simulink model "gm_MATE_HDLsolver_myFirstCircuit"  (R2024b)
settings: Solver=FixedStepDiscrete  StartTime=0.0  StopTime=0.05  FixedStep=6.02409638554217e-09  MaxStep=100e-6  RelTol=1e-4
PostLoadFcn:
  | Ts=1e-6; nb_sw=3; nb_lc=2;nb_r=1;nb_src=1; nb_out=3; rL=1.2;rC=100;L=1e-3; C=1e-5; LpejoSw=1e-6;h=Ts; MAX_INPUTS=16;
  | MAX_OUTPUTS=16;
  | MAX_SWITCHES=8;
  | MAX_INPUTS=16;
InitFcn:
  | Ts=1e-6; nb_sw=3; nb_lc=2;nb_r=1;nb_src=1; nb_out=3; rL=1.2;rC=100;L=1e-3; C=1e-5; LpejoSw=1e-6;h=Ts; MAX_INPUTS=16;
  | MAX_OUTPUTS=16;
  | MAX_SWITCHES=8;
  | MAX_INPUTS=16;
undefined symbols (not defined in the file or in its folder): MATE_SOC
libraries: fl_lib x31, nesl_utility x13, hdlmdlgenlib x10, simetranss x5, simulink x4, hdlsllib x3, ee_lib x2, eeGeneralControl x1
(part 6 of 8)

== system gm_MATE_HDLsolver_myFirstCircuit/ForFPGA/mul_Dot Product13_dotp_7 ==
  In1 : Inport
  In2 : Inport  Port=2
  mul_Dot Product13_dotp_7 : Product  Inputs=**  OutDataTypeStr=single  SampleTime=6.02409638554217e-09
  mul_Dot Product13_dotp_7_pd1 : Delay  DelayLength=6
  Out1 : Outport
  wires:
  In1/1 -> mul_Dot Product13_dotp_7/1
  In2/1 -> mul_Dot Product13_dotp_7/2
  mul_Dot Product13_dotp_7/1 -> mul_Dot Product13_dotp_7_pd1/1
  mul_Dot Product13_dotp_7_pd1/1 -> Out1/1

== system gm_MATE_HDLsolver_myFirstCircuit/ForFPGA/mul_Dot Product13_dotp_8 ==
  In1 : Inport
  In2 : Inport  Port=2
  mul_Dot Product13_dotp_8 : Product  Inputs=**  OutDataTypeStr=single  SampleTime=6.02409638554217e-09
  mul_Dot Product13_dotp_8_pd1 : Delay  DelayLength=6
  Out1 : Outport
  wires:
  In1/1 -> mul_Dot Product13_dotp_8/1
  In2/1 -> mul_Dot Product13_dotp_8/2
  mul_Dot Product13_dotp_8/1 -> mul_Dot Product13_dotp_8_pd1/1
  mul_Dot Product13_dotp_8_pd1/1 -> Out1/1

== system gm_MATE_HDLsolver_myFirstCircuit/ForFPGA/mul_Dot Product13_dotp_9 ==
  In1 : Inport
  In2 : Inport  Port=2
  mul_Dot Product13_dotp_9 : Product  Inputs=**  OutDataTypeStr=single  SampleTime=6.02409638554217e-09
  mul_Dot Product13_dotp_9_pd1 : Delay  DelayLength=6
  Out1 : Outport
  wires:
  In1/1 -> mul_Dot Product13_dotp_9/1
  In2/1 -> mul_Dot Product13_dotp_9/2
  mul_Dot Product13_dotp_9/1 -> mul_Dot Product13_dotp_9_pd1/1
  mul_Dot Product13_dotp_9_pd1/1 -> Out1/1

== system gm_MATE_HDLsolver_myFirstCircuit/ForFPGA/mul_Dot Product14_dotp_0 ==
  In1 : Inport
  In2 : Inport  Port=2
  mul_Dot Product14_dotp_0 : Product  Inputs=**  OutDataTypeStr=single  SampleTime=6.02409638554217e-09
  mul_Dot Product14_dotp_0_pd1 : Delay  DelayLength=6
  Out1 : Outport
  wires:
  In1/1 -> mul_Dot Product14_dotp_0/1
  In2/1 -> mul_Dot Product14_dotp_0/2
  mul_Dot Product14_dotp_0/1 -> mul_Dot Product14_dotp_0_pd1/1
  mul_Dot Product14_dotp_0_pd1/1 -> Out1/1

== system gm_MATE_HDLsolver_myFirstCircuit/ForFPGA/mul_Dot Product14_dotp_1 ==
  In1 : Inport
  In2 : Inport  Port=2
  mul_Dot Product14_dotp_1 : Product  Inputs=**  OutDataTypeStr=single  SampleTime=6.02409638554217e-09
  mul_Dot Product14_dotp_1_pd1 : Delay  DelayLength=6
  Out1 : Outport
  wires:
  In1/1 -> mul_Dot Product14_dotp_1/1
  In2/1 -> mul_Dot Product14_dotp_1/2
  mul_Dot Product14_dotp_1/1 -> mul_Dot Product14_dotp_1_pd1/1
  mul_Dot Product14_dotp_1_pd1/1 -> Out1/1

== system gm_MATE_HDLsolver_myFirstCircuit/ForFPGA/mul_Dot Product14_dotp_10 ==
  In1 : Inport
  In2 : Inport  Port=2
  mul_Dot Product14_dotp_10 : Product  Inputs=**  OutDataTypeStr=single  SampleTime=6.02409638554217e-09
  mul_Dot Product14_dotp_10_pd1 : Delay  DelayLength=6
  Out1 : Outport
  wires:
  In1/1 -> mul_Dot Product14_dotp_10/1
  In2/1 -> mul_Dot Product14_dotp_10/2
  mul_Dot Product14_dotp_10/1 -> mul_Dot Product14_dotp_10_pd1/1
  mul_Dot Product14_dotp_10_pd1/1 -> Out1/1

== system gm_MATE_HDLsolver_myFirstCircuit/ForFPGA/mul_Dot Product14_dotp_11 ==
  In1 : Inport
  In2 : Inport  Port=2
  mul_Dot Product14_dotp_11 : Product  Inputs=**  OutDataTypeStr=single  SampleTime=6.02409638554217e-09
  mul_Dot Product14_dotp_11_pd1 : Delay  DelayLength=6
  Out1 : Outport
  wires:
  In1/1 -> mul_Dot Product14_dotp_11/1
  In2/1 -> mul_Dot Product14_dotp_11/2
  mul_Dot Product14_dotp_11/1 -> mul_Dot Product14_dotp_11_pd1/1
  mul_Dot Product14_dotp_11_pd1/1 -> Out1/1

== system gm_MATE_HDLsolver_myFirstCircuit/ForFPGA/mul_Dot Product14_dotp_12 ==
  In1 : Inport
  In2 : Inport  Port=2
  mul_Dot Product14_dotp_12 : Product  Inputs=**  OutDataTypeStr=single  SampleTime=6.02409638554217e-09
  mul_Dot Product14_dotp_12_pd1 : Delay  DelayLength=6
  Out1 : Outport
  wires:
  In1/1 -> mul_Dot Product14_dotp_12/1
  In2/1 -> mul_Dot Product14_dotp_12/2
  mul_Dot Product14_dotp_12/1 -> mul_Dot Product14_dotp_12_pd1/1
  mul_Dot Product14_dotp_12_pd1/1 -> Out1/1

== system gm_MATE_HDLsolver_myFirstCircuit/ForFPGA/mul_Dot Product14_dotp_13 ==
  In1 : Inport
  In2 : Inport  Port=2
  mul_Dot Product14_dotp_13 : Product  Inputs=**  OutDataTypeStr=single  SampleTime=6.02409638554217e-09
  mul_Dot Product14_dotp_13_pd1 : Delay  DelayLength=6
  Out1 : Outport
  wires:
  In1/1 -> mul_Dot Product14_dotp_13/1
  In2/1 -> mul_Dot Product14_dotp_13/2
  mul_Dot Product14_dotp_13/1 -> mul_Dot Product14_dotp_13_pd1/1
  mul_Dot Product14_dotp_13_pd1/1 -> Out1/1

== system gm_MATE_HDLsolver_myFirstCircuit/ForFPGA/mul_Dot Product14_dotp_14 ==
  In1 : Inport
  In2 : Inport  Port=2
  mul_Dot Product14_dotp_14 : Product  Inputs=**  OutDataTypeStr=single  SampleTime=6.02409638554217e-09
  mul_Dot Product14_dotp_14_pd1 : Delay  DelayLength=6
  Out1 : Outport
  wires:
  In1/1 -> mul_Dot Product14_dotp_14/1
  In2/1 -> mul_Dot Product14_dotp_14/2
  mul_Dot Product14_dotp_14/1 -> mul_Dot Product14_dotp_14_pd1/1
  mul_Dot Product14_dotp_14_pd1/1 -> Out1/1

== system gm_MATE_HDLsolver_myFirstCircuit/ForFPGA/mul_Dot Product14_dotp_15 ==
  In1 : Inport
  In2 : Inport  Port=2
  mul_Dot Product14_dotp_15 : Product  Inputs=**  OutDataTypeStr=single  SampleTime=6.02409638554217e-09
  mul_Dot Product14_dotp_15_pd1 : Delay  DelayLength=6
  Out1 : Outport
  wires:
  In1/1 -> mul_Dot Product14_dotp_15/1
  In2/1 -> mul_Dot Product14_dotp_15/2
  mul_Dot Product14_dotp_15/1 -> mul_Dot Product14_dotp_15_pd1/1
  mul_Dot Product14_dotp_15_pd1/1 -> Out1/1

== system gm_MATE_HDLsolver_myFirstCircuit/ForFPGA/mul_Dot Product14_dotp_2 ==
  In1 : Inport
  In2 : Inport  Port=2
  mul_Dot Product14_dotp_2 : Product  Inputs=**  OutDataTypeStr=single  SampleTime=6.02409638554217e-09
  mul_Dot Product14_dotp_2_pd1 : Delay  DelayLength=6
  Out1 : Outport
  wires:
  In1/1 -> mul_Dot Product14_dotp_2/1
  In2/1 -> mul_Dot Product14_dotp_2/2
  mul_Dot Product14_dotp_2/1 -> mul_Dot Product14_dotp_2_pd1/1
  mul_Dot Product14_dotp_2_pd1/1 -> Out1/1

== system gm_MATE_HDLsolver_myFirstCircuit/ForFPGA/mul_Dot Product14_dotp_3 ==
  In1 : Inport
  In2 : Inport  Port=2
  mul_Dot Product14_dotp_3 : Product  Inputs=**  OutDataTypeStr=single  SampleTime=6.02409638554217e-09
  mul_Dot Product14_dotp_3_pd1 : Delay  DelayLength=6
  Out1 : Outport
  wires:
  In1/1 -> mul_Dot Product14_dotp_3/1
  In2/1 -> mul_Dot Product14_dotp_3/2
  mul_Dot Product14_dotp_3/1 -> mul_Dot Product14_dotp_3_pd1/1
  mul_Dot Product14_dotp_3_pd1/1 -> Out1/1

== system gm_MATE_HDLsolver_myFirstCircuit/ForFPGA/mul_Dot Product14_dotp_4 ==
  In1 : Inport
  In2 : Inport  Port=2
  mul_Dot Product14_dotp_4 : Product  Inputs=**  OutDataTypeStr=single  SampleTime=6.02409638554217e-09
  mul_Dot Product14_dotp_4_pd1 : Delay  DelayLength=6
  Out1 : Outport
  wires:
  In1/1 -> mul_Dot Product14_dotp_4/1
  In2/1 -> mul_Dot Product14_dotp_4/2
  mul_Dot Product14_dotp_4/1 -> mul_Dot Product14_dotp_4_pd1/1
  mul_Dot Product14_dotp_4_pd1/1 -> Out1/1

== system gm_MATE_HDLsolver_myFirstCircuit/ForFPGA/mul_Dot Product14_dotp_5 ==
  In1 : Inport
  In2 : Inport  Port=2
  mul_Dot Product14_dotp_5 : Product  Inputs=**  OutDataTypeStr=single  SampleTime=6.02409638554217e-09
  mul_Dot Product14_dotp_5_pd1 : Delay  DelayLength=6
  Out1 : Outport
  wires:
  In1/1 -> mul_Dot Product14_dotp_5/1
  In2/1 -> mul_Dot Product14_dotp_5/2
  mul_Dot Product14_dotp_5/1 -> mul_Dot Product14_dotp_5_pd1/1
  mul_Dot Product14_dotp_5_pd1/1 -> Out1/1

== system gm_MATE_HDLsolver_myFirstCircuit/ForFPGA/mul_Dot Product14_dotp_6 ==
  In1 : Inport
  In2 : Inport  Port=2
  mul_Dot Product14_dotp_6 : Product  Inputs=**  OutDataTypeStr=single  SampleTime=6.02409638554217e-09
  mul_Dot Product14_dotp_6_pd1 : Delay  DelayLength=6
  Out1 : Outport
  wires:
  In1/1 -> mul_Dot Product14_dotp_6/1
  In2/1 -> mul_Dot Product14_dotp_6/2
  mul_Dot Product14_dotp_6/1 -> mul_Dot Product14_dotp_6_pd1/1
  mul_Dot Product14_dotp_6_pd1/1 -> Out1/1

== system gm_MATE_HDLsolver_myFirstCircuit/ForFPGA/mul_Dot Product14_dotp_7 ==
  In1 : Inport
  In2 : Inport  Port=2
  mul_Dot Product14_dotp_7 : Product  Inputs=**  OutDataTypeStr=single  SampleTime=6.02409638554217e-09
  mul_Dot Product14_dotp_7_pd1 : Delay  DelayLength=6
  Out1 : Outport
  wires:
  In1/1 -> mul_Dot Product14_dotp_7/1
  In2/1 -> mul_Dot Product14_dotp_7/2
  mul_Dot Product14_dotp_7/1 -> mul_Dot Product14_dotp_7_pd1/1
  mul_Dot Product14_dotp_7_pd1/1 -> Out1/1

== system gm_MATE_HDLsolver_myFirstCircuit/ForFPGA/mul_Dot Product14_dotp_8 ==
  In1 : Inport
  In2 : Inport  Port=2
  mul_Dot Product14_dotp_8 : Product  Inputs=**  OutDataTypeStr=single  SampleTime=6.02409638554217e-09
  mul_Dot Product14_dotp_8_pd1 : Delay  DelayLength=6
  Out1 : Outport
  wires:
  In1/1 -> mul_Dot Product14_dotp_8/1
  In2/1 -> mul_Dot Product14_dotp_8/2
  mul_Dot Product14_dotp_8/1 -> mul_Dot Product14_dotp_8_pd1/1
  mul_Dot Product14_dotp_8_pd1/1 -> Out1/1

== system gm_MATE_HDLsolver_myFirstCircuit/ForFPGA/mul_Dot Product14_dotp_9 ==
  In1 : Inport
  In2 : Inport  Port=2
  mul_Dot Product14_dotp_9 : Product  Inputs=**  OutDataTypeStr=single  SampleTime=6.02409638554217e-09
  mul_Dot Product14_dotp_9_pd1 : Delay  DelayLength=6
  Out1 : Outport
  wires:
  In1/1 -> mul_Dot Product14_dotp_9/1
  In2/1 -> mul_Dot Product14_dotp_9/2
  mul_Dot Product14_dotp_9/1 -> mul_Dot Product14_dotp_9_pd1/1
  mul_Dot Product14_dotp_9_pd1/1 -> Out1/1

== system gm_MATE_HDLsolver_myFirstCircuit/ForFPGA/mul_Dot Product15_dotp_0 ==
  In1 : Inport
  In2 : Inport  Port=2
  mul_Dot Product15_dotp_0 : Product  Inputs=**  OutDataTypeStr=single  SampleTime=6.02409638554217e-09
  mul_Dot Product15_dotp_0_pd1 : Delay  DelayLength=6
  Out1 : Outport
  wires:
  In1/1 -> mul_Dot Product15_dotp_0/1
  In2/1 -> mul_Dot Product15_dotp_0/2
  mul_Dot Product15_dotp_0/1 -> mul_Dot Product15_dotp_0_pd1/1
  mul_Dot Product15_dotp_0_pd1/1 -> Out1/1

== system gm_MATE_HDLsolver_myFirstCircuit/ForFPGA/mul_Dot Product15_dotp_1 ==
  In1 : Inport
  In2 : Inport  Port=2
  mul_Dot Product15_dotp_1 : Product  Inputs=**  OutDataTypeStr=single  SampleTime=6.02409638554217e-09
  mul_Dot Product15_dotp_1_pd1 : Delay  DelayLength=6
  Out1 : Outport
  wires:
  In1/1 -> mul_Dot Product15_dotp_1/1
  In2/1 -> mul_Dot Product15_dotp_1/2
  mul_Dot Product15_dotp_1/1 -> mul_Dot Product15_dotp_1_pd1/1
  mul_Dot Product15_dotp_1_pd1/1 -> Out1/1

== system gm_MATE_HDLsolver_myFirstCircuit/ForFPGA/mul_Dot Product15_dotp_10 ==
  In1 : Inport
  In2 : Inport  Port=2
  mul_Dot Product15_dotp_10 : Product  Inputs=**  OutDataTypeStr=single  SampleTime=6.02409638554217e-09
  mul_Dot Product15_dotp_10_pd1 : Delay  DelayLength=6
  Out1 : Outport
  wires:
  In1/1 -> mul_Dot Product15_dotp_10/1
  In2/1 -> mul_Dot Product15_dotp_10/2
  mul_Dot Product15_dotp_10/1 -> mul_Dot Product15_dotp_10_pd1/1
  mul_Dot Product15_dotp_10_pd1/1 -> Out1/1

== system gm_MATE_HDLsolver_myFirstCircuit/ForFPGA/mul_Dot Product15_dotp_11 ==
  In1 : Inport
  In2 : Inport  Port=2
  mul_Dot Product15_dotp_11 : Product  Inputs=**  OutDataTypeStr=single  SampleTime=6.02409638554217e-09
  mul_Dot Product15_dotp_11_pd1 : Delay  DelayLength=6
  Out1 : Outport
  wires:
  In1/1 -> mul_Dot Product15_dotp_11/1
  In2/1 -> mul_Dot Product15_dotp_11/2
  mul_Dot Product15_dotp_11/1 -> mul_Dot Product15_dotp_11_pd1/1
  mul_Dot Product15_dotp_11_pd1/1 -> Out1/1

== system gm_MATE_HDLsolver_myFirstCircuit/ForFPGA/mul_Dot Product15_dotp_12 ==
  In1 : Inport
  In2 : Inport  Port=2
  mul_Dot Product15_dotp_12 : Product  Inputs=**  OutDataTypeStr=single  SampleTime=6.02409638554217e-09
  mul_Dot Product15_dotp_12_pd1 : Delay  DelayLength=6
  Out1 : Outport
  wires:
  In1/1 -> mul_Dot Product15_dotp_12/1
  In2/1 -> mul_Dot Product15_dotp_12/2
  mul_Dot Product15_dotp_12/1 -> mul_Dot Product15_dotp_12_pd1/1
  mul_Dot Product15_dotp_12_pd1/1 -> Out1/1

== system gm_MATE_HDLsolver_myFirstCircuit/ForFPGA/mul_Dot Product15_dotp_13 ==
  In1 : Inport
  In2 : Inport  Port=2
  mul_Dot Product15_dotp_13 : Product  Inputs=**  OutDataTypeStr=single  SampleTime=6.02409638554217e-09
  mul_Dot Product15_dotp_13_pd1 : Delay  DelayLength=6
  Out1 : Outport
  wires:
  In1/1 -> mul_Dot Product15_dotp_13/1
  In2/1 -> mul_Dot Product15_dotp_13/2
  mul_Dot Product15_dotp_13/1 -> mul_Dot Product15_dotp_13_pd1/1
  mul_Dot Product15_dotp_13_pd1/1 -> Out1/1

== system gm_MATE_HDLsolver_myFirstCircuit/ForFPGA/mul_Dot Product15_dotp_14 ==
  In1 : Inport
  In2 : Inport  Port=2
  mul_Dot Product15_dotp_14 : Product  Inputs=**  OutDataTypeStr=single  SampleTime=6.02409638554217e-09
  mul_Dot Product15_dotp_14_pd1 : Delay  DelayLength=6
  Out1 : Outport
  wires:
  In1/1 -> mul_Dot Product15_dotp_14/1
  In2/1 -> mul_Dot Product15_dotp_14/2
  mul_Dot Product15_dotp_14/1 -> mul_Dot Product15_dotp_14_pd1/1
  mul_Dot Product15_dotp_14_pd1/1 -> Out1/1

== system gm_MATE_HDLsolver_myFirstCircuit/ForFPGA/mul_Dot Product15_dotp_15 ==
  In1 : Inport
  In2 : Inport  Port=2
  mul_Dot Product15_dotp_15 : Product  Inputs=**  OutDataTypeStr=single  SampleTime=6.02409638554217e-09
  mul_Dot Product15_dotp_15_pd1 : Delay  DelayLength=6
  Out1 : Outport
  wires:
  In1/1 -> mul_Dot Product15_dotp_15/1
  In2/1 -> mul_Dot Product15_dotp_15/2
  mul_Dot Product15_dotp_15/1 -> mul_Dot Product15_dotp_15_pd1/1
  mul_Dot Product15_dotp_15_pd1/1 -> Out1/1

== system gm_MATE_HDLsolver_myFirstCircuit/ForFPGA/mul_Dot Product15_dotp_2 ==
  In1 : Inport
  In2 : Inport  Port=2
  mul_Dot Product15_dotp_2 : Product  Inputs=**  OutDataTypeStr=single  SampleTime=6.02409638554217e-09
  mul_Dot Product15_dotp_2_pd1 : Delay  DelayLength=6
  Out1 : Outport
  wires:
  In1/1 -> mul_Dot Product15_dotp_2/1
  In2/1 -> mul_Dot Product15_dotp_2/2
  mul_Dot Product15_dotp_2/1 -> mul_Dot Product15_dotp_2_pd1/1
  mul_Dot Product15_dotp_2_pd1/1 -> Out1/1

== system gm_MATE_HDLsolver_myFirstCircuit/ForFPGA/mul_Dot Product15_dotp_3 ==
  In1 : Inport
  In2 : Inport  Port=2
  mul_Dot Product15_dotp_3 : Product  Inputs=**  OutDataTypeStr=single  SampleTime=6.02409638554217e-09
  mul_Dot Product15_dotp_3_pd1 : Delay  DelayLength=6
  Out1 : Outport
  wires:
  In1/1 -> mul_Dot Product15_dotp_3/1
  In2/1 -> mul_Dot Product15_dotp_3/2
  mul_Dot Product15_dotp_3/1 -> mul_Dot Product15_dotp_3_pd1/1
  mul_Dot Product15_dotp_3_pd1/1 -> Out1/1

== system gm_MATE_HDLsolver_myFirstCircuit/ForFPGA/mul_Dot Product15_dotp_4 ==
  In1 : Inport
  In2 : Inport  Port=2
  mul_Dot Product15_dotp_4 : Product  Inputs=**  OutDataTypeStr=single  SampleTime=6.02409638554217e-09
  mul_Dot Product15_dotp_4_pd1 : Delay  DelayLength=6
  Out1 : Outport
  wires:
  In1/1 -> mul_Dot Product15_dotp_4/1
  In2/1 -> mul_Dot Product15_dotp_4/2
  mul_Dot Product15_dotp_4/1 -> mul_Dot Product15_dotp_4_pd1/1
  mul_Dot Product15_dotp_4_pd1/1 -> Out1/1

== system gm_MATE_HDLsolver_myFirstCircuit/ForFPGA/mul_Dot Product15_dotp_5 ==
  In1 : Inport
  In2 : Inport  Port=2
  mul_Dot Product15_dotp_5 : Product  Inputs=**  OutDataTypeStr=single  SampleTime=6.02409638554217e-09
  mul_Dot Product15_dotp_5_pd1 : Delay  DelayLength=6
  Out1 : Outport
  wires:
  In1/1 -> mul_Dot Product15_dotp_5/1
  In2/1 -> mul_Dot Product15_dotp_5/2
  mul_Dot Product15_dotp_5/1 -> mul_Dot Product15_dotp_5_pd1/1
  mul_Dot Product15_dotp_5_pd1/1 -> Out1/1

== system gm_MATE_HDLsolver_myFirstCircuit/ForFPGA/mul_Dot Product15_dotp_6 ==
  In1 : Inport
  In2 : Inport  Port=2
  mul_Dot Product15_dotp_6 : Product  Inputs=**  OutDataTypeStr=single  SampleTime=6.02409638554217e-09
  mul_Dot Product15_dotp_6_pd1 : Delay  DelayLength=6
  Out1 : Outport
  wires:
  In1/1 -> mul_Dot Product15_dotp_6/1
  In2/1 -> mul_Dot Product15_dotp_6/2
  mul_Dot Product15_dotp_6/1 -> mul_Dot Product15_dotp_6_pd1/1
  mul_Dot Product15_dotp_6_pd1/1 -> Out1/1

== system gm_MATE_HDLsolver_myFirstCircuit/ForFPGA/mul_Dot Product15_dotp_7 ==
  In1 : Inport
  In2 : Inport  Port=2
  mul_Dot Product15_dotp_7 : Product  Inputs=**  OutDataTypeStr=single  SampleTime=6.02409638554217e-09
  mul_Dot Product15_dotp_7_pd1 : Delay  DelayLength=6
  Out1 : Outport
  wires:
  In1/1 -> mul_Dot Product15_dotp_7/1
  In2/1 -> mul_Dot Product15_dotp_7/2
  mul_Dot Product15_dotp_7/1 -> mul_Dot Product15_dotp_7_pd1/1
  mul_Dot Product15_dotp_7_pd1/1 -> Out1/1

== system gm_MATE_HDLsolver_myFirstCircuit/ForFPGA/mul_Dot Product15_dotp_8 ==
  In1 : Inport
  In2 : Inport  Port=2
  mul_Dot Product15_dotp_8 : Product  Inputs=**  OutDataTypeStr=single  SampleTime=6.02409638554217e-09
  mul_Dot Product15_dotp_8_pd1 : Delay  DelayLength=6
  Out1 : Outport
  wires:
  In1/1 -> mul_Dot Product15_dotp_8/1
  In2/1 -> mul_Dot Product15_dotp_8/2
  mul_Dot Product15_dotp_8/1 -> mul_Dot Product15_dotp_8_pd1/1
  mul_Dot Product15_dotp_8_pd1/1 -> Out1/1

== system gm_MATE_HDLsolver_myFirstCircuit/ForFPGA/mul_Dot Product15_dotp_9 ==
  In1 : Inport
  In2 : Inport  Port=2
  mul_Dot Product15_dotp_9 : Product  Inputs=**  OutDataTypeStr=single  SampleTime=6.02409638554217e-09
  mul_Dot Product15_dotp_9_pd1 : Delay  DelayLength=6
  Out1 : Outport
  wires:
  In1/1 -> mul_Dot Product15_dotp_9/1
  In2/1 -> mul_Dot Product15_dotp_9/2
  mul_Dot Product15_dotp_9/1 -> mul_Dot Product15_dotp_9_pd1/1
  mul_Dot Product15_dotp_9_pd1/1 -> Out1/1

== system gm_MATE_HDLsolver_myFirstCircuit/ForFPGA/mul_Dot Product1_dotp_0 ==
  In1 : Inport
  In2 : Inport  Port=2
  mul_Dot Product1_dotp_0 : Product  Inputs=**  OutDataTypeStr=single  SampleTime=6.02409638554217e-09
  mul_Dot Product1_dotp_0_pd1 : Delay  DelayLength=6
  Out1 : Outport
  wires:
  In1/1 -> mul_Dot Product1_dotp_0/1
  In2/1 -> mul_Dot Product1_dotp_0/2
  mul_Dot Product1_dotp_0/1 -> mul_Dot Product1_dotp_0_pd1/1
  mul_Dot Product1_dotp_0_pd1/1 -> Out1/1

== system gm_MATE_HDLsolver_myFirstCircuit/ForFPGA/mul_Dot Product1_dotp_1 ==
  In1 : Inport
  In2 : Inport  Port=2
  mul_Dot Product1_dotp_1 : Product  Inputs=**  OutDataTypeStr=single  SampleTime=6.02409638554217e-09
  mul_Dot Product1_dotp_1_pd1 : Delay  DelayLength=6
  Out1 : Outport
  wires:
  In1/1 -> mul_Dot Product1_dotp_1/1
  In2/1 -> mul_Dot Product1_dotp_1/2
  mul_Dot Product1_dotp_1/1 -> mul_Dot Product1_dotp_1_pd1/1
  mul_Dot Product1_dotp_1_pd1/1 -> Out1/1

== system gm_MATE_HDLsolver_myFirstCircuit/ForFPGA/mul_Dot Product1_dotp_10 ==
  In1 : Inport
  In2 : Inport  Port=2
  mul_Dot Product1_dotp_10 : Product  Inputs=**  OutDataTypeStr=single  SampleTime=6.02409638554217e-09
  mul_Dot Product1_dotp_10_pd1 : Delay  DelayLength=6
  Out1 : Outport
  wires:
  In1/1 -> mul_Dot Product1_dotp_10/1
  In2/1 -> mul_Dot Product1_dotp_10/2
  mul_Dot Product1_dotp_10/1 -> mul_Dot Product1_dotp_10_pd1/1
  mul_Dot Product1_dotp_10_pd1/1 -> Out1/1

== system gm_MATE_HDLsolver_myFirstCircuit/ForFPGA/mul_Dot Product1_dotp_11 ==
  In1 : Inport
  In2 : Inport  Port=2
  mul_Dot Product1_dotp_11 : Product  Inputs=**  OutDataTypeStr=single  SampleTime=6.02409638554217e-09
  mul_Dot Product1_dotp_11_pd1 : Delay  DelayLength=6
  Out1 : Outport
  wires:
  In1/1 -> mul_Dot Product1_dotp_11/1
  In2/1 -> mul_Dot Product1_dotp_11/2
  mul_Dot Product1_dotp_11/1 -> mul_Dot Product1_dotp_11_pd1/1
  mul_Dot Product1_dotp_11_pd1/1 -> Out1/1

== system gm_MATE_HDLsolver_myFirstCircuit/ForFPGA/mul_Dot Product1_dotp_12 ==
  In1 : Inport
  In2 : Inport  Port=2
  mul_Dot Product1_dotp_12 : Product  Inputs=**  OutDataTypeStr=single  SampleTime=6.02409638554217e-09
  mul_Dot Product1_dotp_12_pd1 : Delay  DelayLength=6
  Out1 : Outport
  wires:
  In1/1 -> mul_Dot Product1_dotp_12/1
  In2/1 -> mul_Dot Product1_dotp_12/2
  mul_Dot Product1_dotp_12/1 -> mul_Dot Product1_dotp_12_pd1/1
  mul_Dot Product1_dotp_12_pd1/1 -> Out1/1

== system gm_MATE_HDLsolver_myFirstCircuit/ForFPGA/mul_Dot Product1_dotp_13 ==
  In1 : Inport
  In2 : Inport  Port=2
  mul_Dot Product1_dotp_13 : Product  Inputs=**  OutDataTypeStr=single  SampleTime=6.02409638554217e-09
  mul_Dot Product1_dotp_13_pd1 : Delay  DelayLength=6
  Out1 : Outport
  wires:
  In1/1 -> mul_Dot Product1_dotp_13/1
  In2/1 -> mul_Dot Product1_dotp_13/2
  mul_Dot Product1_dotp_13/1 -> mul_Dot Product1_dotp_13_pd1/1
  mul_Dot Product1_dotp_13_pd1/1 -> Out1/1

== system gm_MATE_HDLsolver_myFirstCircuit/ForFPGA/mul_Dot Product1_dotp_14 ==
  In1 : Inport
  In2 : Inport  Port=2
  mul_Dot Product1_dotp_14 : Product  Inputs=**  OutDataTypeStr=single  SampleTime=6.02409638554217e-09
  mul_Dot Product1_dotp_14_pd1 : Delay  DelayLength=6
  Out1 : Outport
  wires:
  In1/1 -> mul_Dot Product1_dotp_14/1
  In2/1 -> mul_Dot Product1_dotp_14/2
  mul_Dot Product1_dotp_14/1 -> mul_Dot Product1_dotp_14_pd1/1
  mul_Dot Product1_dotp_14_pd1/1 -> Out1/1

== system gm_MATE_HDLsolver_myFirstCircuit/ForFPGA/mul_Dot Product1_dotp_15 ==
  In1 : Inport
  In2 : Inport  Port=2
  mul_Dot Product1_dotp_15 : Product  Inputs=**  OutDataTypeStr=single  SampleTime=6.02409638554217e-09
  mul_Dot Product1_dotp_15_pd1 : Delay  DelayLength=6
  Out1 : Outport
  wires:
  In1/1 -> mul_Dot Product1_dotp_15/1
  In2/1 -> mul_Dot Product1_dotp_15/2
  mul_Dot Product1_dotp_15/1 -> mul_Dot Product1_dotp_15_pd1/1
  mul_Dot Product1_dotp_15_pd1/1 -> Out1/1

== system gm_MATE_HDLsolver_myFirstCircuit/ForFPGA/mul_Dot Product1_dotp_2 ==
  In1 : Inport
  In2 : Inport  Port=2
  mul_Dot Product1_dotp_2 : Product  Inputs=**  OutDataTypeStr=single  SampleTime=6.02409638554217e-09
  mul_Dot Product1_dotp_2_pd1 : Delay  DelayLength=6
  Out1 : Outport
  wires:
  In1/1 -> mul_Dot Product1_dotp_2/1
  In2/1 -> mul_Dot Product1_dotp_2/2
  mul_Dot Product1_dotp_2/1 -> mul_Dot Product1_dotp_2_pd1/1
  mul_Dot Product1_dotp_2_pd1/1 -> Out1/1

== system gm_MATE_HDLsolver_myFirstCircuit/ForFPGA/mul_Dot Product1_dotp_3 ==
  In1 : Inport
  In2 : Inport  Port=2
  mul_Dot Product1_dotp_3 : Product  Inputs=**  OutDataTypeStr=single  SampleTime=6.02409638554217e-09
  mul_Dot Product1_dotp_3_pd1 : Delay  DelayLength=6
  Out1 : Outport
  wires:
  In1/1 -> mul_Dot Product1_dotp_3/1
  In2/1 -> mul_Dot Product1_dotp_3/2
  mul_Dot Product1_dotp_3/1 -> mul_Dot Product1_dotp_3_pd1/1
  mul_Dot Product1_dotp_3_pd1/1 -> Out1/1

== system gm_MATE_HDLsolver_myFirstCircuit/ForFPGA/mul_Dot Product1_dotp_4 ==
  In1 : Inport
  In2 : Inport  Port=2
  mul_Dot Product1_dotp_4 : Product  Inputs=**  OutDataTypeStr=single  SampleTime=6.02409638554217e-09
  mul_Dot Product1_dotp_4_pd1 : Delay  DelayLength=6
  Out1 : Outport
  wires:
  In1/1 -> mul_Dot Product1_dotp_4/1
  In2/1 -> mul_Dot Product1_dotp_4/2
  mul_Dot Product1_dotp_4/1 -> mul_Dot Product1_dotp_4_pd1/1
  mul_Dot Product1_dotp_4_pd1/1 -> Out1/1

== system gm_MATE_HDLsolver_myFirstCircuit/ForFPGA/mul_Dot Product1_dotp_5 ==
  In1 : Inport
  In2 : Inport  Port=2
  mul_Dot Product1_dotp_5 : Product  Inputs=**  OutDataTypeStr=single  SampleTime=6.02409638554217e-09
  mul_Dot Product1_dotp_5_pd1 : Delay  DelayLength=6
  Out1 : Outport
  wires:
  In1/1 -> mul_Dot Product1_dotp_5/1
  In2/1 -> mul_Dot Product1_dotp_5/2
  mul_Dot Product1_dotp_5/1 -> mul_Dot Product1_dotp_5_pd1/1
  mul_Dot Product1_dotp_5_pd1/1 -> Out1/1

== system gm_MATE_HDLsolver_myFirstCircuit/ForFPGA/mul_Dot Product1_dotp_6 ==
  In1 : Inport
  In2 : Inport  Port=2
  mul_Dot Product1_dotp_6 : Product  Inputs=**  OutDataTypeStr=single  SampleTime=6.02409638554217e-09
  mul_Dot Product1_dotp_6_pd1 : Delay  DelayLength=6
  Out1 : Outport
  wires:
  In1/1 -> mul_Dot Product1_dotp_6/1
  In2/1 -> mul_Dot Product1_dotp_6/2
  mul_Dot Product1_dotp_6/1 -> mul_Dot Product1_dotp_6_pd1/1
  mul_Dot Product1_dotp_6_pd1/1 -> Out1/1

== system gm_MATE_HDLsolver_myFirstCircuit/ForFPGA/mul_Dot Product1_dotp_7 ==
  In1 : Inport
  In2 : Inport  Port=2
  mul_Dot Product1_dotp_7 : Product  Inputs=**  OutDataTypeStr=single  SampleTime=6.02409638554217e-09
  mul_Dot Product1_dotp_7_pd1 : Delay  DelayLength=6
  Out1 : Outport
  wires:
  In1/1 -> mul_Dot Product1_dotp_7/1
  In2/1 -> mul_Dot Product1_dotp_7/2
  mul_Dot Product1_dotp_7/1 -> mul_Dot Product1_dotp_7_pd1/1
  mul_Dot Product1_dotp_7_pd1/1 -> Out1/1

== system gm_MATE_HDLsolver_myFirstCircuit/ForFPGA/mul_Dot Product1_dotp_8 ==
  In1 : Inport
  In2 : Inport  Port=2
  mul_Dot Product1_dotp_8 : Product  Inputs=**  OutDataTypeStr=single  SampleTime=6.02409638554217e-09
  mul_Dot Product1_dotp_8_pd1 : Delay  DelayLength=6
  Out1 : Outport
  wires:
  In1/1 -> mul_Dot Product1_dotp_8/1
  In2/1 -> mul_Dot Product1_dotp_8/2
  mul_Dot Product1_dotp_8/1 -> mul_Dot Product1_dotp_8_pd1/1
  mul_Dot Product1_dotp_8_pd1/1 -> Out1/1

== system gm_MATE_HDLsolver_myFirstCircuit/ForFPGA/mul_Dot Product1_dotp_9 ==
  In1 : Inport
  In2 : Inport  Port=2
  mul_Dot Product1_dotp_9 : Product  Inputs=**  OutDataTypeStr=single  SampleTime=6.02409638554217e-09
  mul_Dot Product1_dotp_9_pd1 : Delay  DelayLength=6
  Out1 : Outport
  wires:
  In1/1 -> mul_Dot Product1_dotp_9/1
  In2/1 -> mul_Dot Product1_dotp_9/2
  mul_Dot Product1_dotp_9/1 -> mul_Dot Product1_dotp_9_pd1/1
  mul_Dot Product1_dotp_9_pd1/1 -> Out1/1

== system gm_MATE_HDLsolver_myFirstCircuit/ForFPGA/mul_Dot Product2_dotp_0 ==
  In1 : Inport
  In2 : Inport  Port=2
  mul_Dot Product2_dotp_0 : Product  Inputs=**  OutDataTypeStr=single  SampleTime=6.02409638554217e-09
  mul_Dot Product2_dotp_0_pd1 : Delay  DelayLength=6
  Out1 : Outport
  wires:
  In1/1 -> mul_Dot Product2_dotp_0/1
  In2/1 -> mul_Dot Product2_dotp_0/2
  mul_Dot Product2_dotp_0/1 -> mul_Dot Product2_dotp_0_pd1/1
  mul_Dot Product2_dotp_0_pd1/1 -> Out1/1

== system gm_MATE_HDLsolver_myFirstCircuit/ForFPGA/mul_Dot Product2_dotp_1 ==
  In1 : Inport
  In2 : Inport  Port=2
  mul_Dot Product2_dotp_1 : Product  Inputs=**  OutDataTypeStr=single  SampleTime=6.02409638554217e-09
  mul_Dot Product2_dotp_1_pd1 : Delay  DelayLength=6
  Out1 : Outport
  wires:
  In1/1 -> mul_Dot Product2_dotp_1/1
  In2/1 -> mul_Dot Product2_dotp_1/2
  mul_Dot Product2_dotp_1/1 -> mul_Dot Product2_dotp_1_pd1/1
  mul_Dot Product2_dotp_1_pd1/1 -> Out1/1

== system gm_MATE_HDLsolver_myFirstCircuit/ForFPGA/mul_Dot Product2_dotp_10 ==
  In1 : Inport
  In2 : Inport  Port=2
  mul_Dot Product2_dotp_10 : Product  Inputs=**  OutDataTypeStr=single  SampleTime=6.02409638554217e-09
  mul_Dot Product2_dotp_10_pd1 : Delay  DelayLength=6
  Out1 : Outport
  wires:
  In1/1 -> mul_Dot Product2_dotp_10/1
  In2/1 -> mul_Dot Product2_dotp_10/2
  mul_Dot Product2_dotp_10/1 -> mul_Dot Product2_dotp_10_pd1/1
  mul_Dot Product2_dotp_10_pd1/1 -> Out1/1

== system gm_MATE_HDLsolver_myFirstCircuit/ForFPGA/mul_Dot Product2_dotp_11 ==
  In1 : Inport
  In2 : Inport  Port=2
  mul_Dot Product2_dotp_11 : Product  Inputs=**  OutDataTypeStr=single  SampleTime=6.02409638554217e-09
  mul_Dot Product2_dotp_11_pd1 : Delay  DelayLength=6
  Out1 : Outport
  wires:
  In1/1 -> mul_Dot Product2_dotp_11/1
  In2/1 -> mul_Dot Product2_dotp_11/2
  mul_Dot Product2_dotp_11/1 -> mul_Dot Product2_dotp_11_pd1/1
  mul_Dot Product2_dotp_11_pd1/1 -> Out1/1

== system gm_MATE_HDLsolver_myFirstCircuit/ForFPGA/mul_Dot Product2_dotp_12 ==
  In1 : Inport
  In2 : Inport  Port=2
  mul_Dot Product2_dotp_12 : Product  Inputs=**  OutDataTypeStr=single  SampleTime=6.02409638554217e-09
  mul_Dot Product2_dotp_12_pd1 : Delay  DelayLength=6
  Out1 : Outport
  wires:
  In1/1 -> mul_Dot Product2_dotp_12/1
  In2/1 -> mul_Dot Product2_dotp_12/2
  mul_Dot Product2_dotp_12/1 -> mul_Dot Product2_dotp_12_pd1/1
  mul_Dot Product2_dotp_12_pd1/1 -> Out1/1

== system gm_MATE_HDLsolver_myFirstCircuit/ForFPGA/mul_Dot Product2_dotp_13 ==
  In1 : Inport
  In2 : Inport  Port=2
  mul_Dot Product2_dotp_13 : Product  Inputs=**  OutDataTypeStr=single  SampleTime=6.02409638554217e-09
  mul_Dot Product2_dotp_13_pd1 : Delay  DelayLength=6
  Out1 : Outport
  wires:
  In1/1 -> mul_Dot Product2_dotp_13/1
  In2/1 -> mul_Dot Product2_dotp_13/2
  mul_Dot Product2_dotp_13/1 -> mul_Dot Product2_dotp_13_pd1/1
  mul_Dot Product2_dotp_13_pd1/1 -> Out1/1

== system gm_MATE_HDLsolver_myFirstCircuit/ForFPGA/mul_Dot Product2_dotp_14 ==
  In1 : Inport
  In2 : Inport  Port=2
  mul_Dot Product2_dotp_14 : Product  Inputs=**  OutDataTypeStr=single  SampleTime=6.02409638554217e-09
  mul_Dot Product2_dotp_14_pd1 : Delay  DelayLength=6
  Out1 : Outport
  wires:
  In1/1 -> mul_Dot Product2_dotp_14/1
  In2/1 -> mul_Dot Product2_dotp_14/2
  mul_Dot Product2_dotp_14/1 -> mul_Dot Product2_dotp_14_pd1/1
  mul_Dot Product2_dotp_14_pd1/1 -> Out1/1

== system gm_MATE_HDLsolver_myFirstCircuit/ForFPGA/mul_Dot Product2_dotp_15 ==
  In1 : Inport
  In2 : Inport  Port=2
  mul_Dot Product2_dotp_15 : Product  Inputs=**  OutDataTypeStr=single  SampleTime=6.02409638554217e-09
  mul_Dot Product2_dotp_15_pd1 : Delay  DelayLength=6
  Out1 : Outport
  wires:
  In1/1 -> mul_Dot Product2_dotp_15/1
  In2/1 -> mul_Dot Product2_dotp_15/2
  mul_Dot Product2_dotp_15/1 -> mul_Dot Product2_dotp_15_pd1/1
  mul_Dot Product2_dotp_15_pd1/1 -> Out1/1

== system gm_MATE_HDLsolver_myFirstCircuit/ForFPGA/mul_Dot Product2_dotp_2 ==
  In1 : Inport
  In2 : Inport  Port=2
  mul_Dot Product2_dotp_2 : Product  Inputs=**  OutDataTypeStr=single  SampleTime=6.02409638554217e-09
  mul_Dot Product2_dotp_2_pd1 : Delay  DelayLength=6
  Out1 : Outport
  wires:
  In1/1 -> mul_Dot Product2_dotp_2/1
  In2/1 -> mul_Dot Product2_dotp_2/2
  mul_Dot Product2_dotp_2/1 -> mul_Dot Product2_dotp_2_pd1/1
  mul_Dot Product2_dotp_2_pd1/1 -> Out1/1

== system gm_MATE_HDLsolver_myFirstCircuit/ForFPGA/mul_Dot Product2_dotp_3 ==
  In1 : Inport
  In2 : Inport  Port=2
  mul_Dot Product2_dotp_3 : Product  Inputs=**  OutDataTypeStr=single  SampleTime=6.02409638554217e-09
  mul_Dot Product2_dotp_3_pd1 : Delay  DelayLength=6
  Out1 : Outport
  wires:
  In1/1 -> mul_Dot Product2_dotp_3/1
  In2/1 -> mul_Dot Product2_dotp_3/2
  mul_Dot Product2_dotp_3/1 -> mul_Dot Product2_dotp_3_pd1/1
  mul_Dot Product2_dotp_3_pd1/1 -> Out1/1

== system gm_MATE_HDLsolver_myFirstCircuit/ForFPGA/mul_Dot Product2_dotp_4 ==
  In1 : Inport
  In2 : Inport  Port=2
  mul_Dot Product2_dotp_4 : Product  Inputs=**  OutDataTypeStr=single  SampleTime=6.02409638554217e-09
  mul_Dot Product2_dotp_4_pd1 : Delay  DelayLength=6
  Out1 : Outport
  wires:
  In1/1 -> mul_Dot Product2_dotp_4/1
  In2/1 -> mul_Dot Product2_dotp_4/2
  mul_Dot Product2_dotp_4/1 -> mul_Dot Product2_dotp_4_pd1/1
  mul_Dot Product2_dotp_4_pd1/1 -> Out1/1

== system gm_MATE_HDLsolver_myFirstCircuit/ForFPGA/mul_Dot Product2_dotp_5 ==
  In1 : Inport
  In2 : Inport  Port=2
  mul_Dot Product2_dotp_5 : Product  Inputs=**  OutDataTypeStr=single  SampleTime=6.02409638554217e-09
  mul_Dot Product2_dotp_5_pd1 : Delay  DelayLength=6
  Out1 : Outport
  wires:
  In1/1 -> mul_Dot Product2_dotp_5/1
  In2/1 -> mul_Dot Product2_dotp_5/2
  mul_Dot Product2_dotp_5/1 -> mul_Dot Product2_dotp_5_pd1/1
  mul_Dot Product2_dotp_5_pd1/1 -> Out1/1

== system gm_MATE_HDLsolver_myFirstCircuit/ForFPGA/mul_Dot Product2_dotp_6 ==
  In1 : Inport
  In2 : Inport  Port=2
  mul_Dot Product2_dotp_6 : Product  Inputs=**  OutDataTypeStr=single  SampleTime=6.02409638554217e-09
  mul_Dot Product2_dotp_6_pd1 : Delay  DelayLength=6
  Out1 : Outport
  wires:
  In1/1 -> mul_Dot Product2_dotp_6/1
  In2/1 -> mul_Dot Product2_dotp_6/2
  mul_Dot Product2_dotp_6/1 -> mul_Dot Product2_dotp_6_pd1/1
  mul_Dot Product2_dotp_6_pd1/1 -> Out1/1

== system gm_MATE_HDLsolver_myFirstCircuit/ForFPGA/mul_Dot Product2_dotp_7 ==
  In1 : Inport
  In2 : Inport  Port=2
  mul_Dot Product2_dotp_7 : Product  Inputs=**  OutDataTypeStr=single  SampleTime=6.02409638554217e-09
  mul_Dot Product2_dotp_7_pd1 : Delay  DelayLength=6
  Out1 : Outport
  wires:
  In1/1 -> mul_Dot Product2_dotp_7/1
  In2/1 -> mul_Dot Product2_dotp_7/2
  mul_Dot Product2_dotp_7/1 -> mul_Dot Product2_dotp_7_pd1/1
  mul_Dot Product2_dotp_7_pd1/1 -> Out1/1

== system gm_MATE_HDLsolver_myFirstCircuit/ForFPGA/mul_Dot Product2_dotp_8 ==
  In1 : Inport
  In2 : Inport  Port=2
  mul_Dot Product2_dotp_8 : Product  Inputs=**  OutDataTypeStr=single  SampleTime=6.02409638554217e-09
  mul_Dot Product2_dotp_8_pd1 : Delay  DelayLength=6
  Out1 : Outport
  wires:
  In1/1 -> mul_Dot Product2_dotp_8/1
  In2/1 -> mul_Dot Product2_dotp_8/2
  mul_Dot Product2_dotp_8/1 -> mul_Dot Product2_dotp_8_pd1/1
  mul_Dot Product2_dotp_8_pd1/1 -> Out1/1

== system gm_MATE_HDLsolver_myFirstCircuit/ForFPGA/mul_Dot Product2_dotp_9 ==
  In1 : Inport
  In2 : Inport  Port=2
  mul_Dot Product2_dotp_9 : Product  Inputs=**  OutDataTypeStr=single  SampleTime=6.02409638554217e-09
  mul_Dot Product2_dotp_9_pd1 : Delay  DelayLength=6
  Out1 : Outport
  wires:
  In1/1 -> mul_Dot Product2_dotp_9/1
  In2/1 -> mul_Dot Product2_dotp_9/2
  mul_Dot Product2_dotp_9/1 -> mul_Dot Product2_dotp_9_pd1/1
  mul_Dot Product2_dotp_9_pd1/1 -> Out1/1

== system gm_MATE_HDLsolver_myFirstCircuit/ForFPGA/mul_Dot Product3_dotp_0 ==
  In1 : Inport
  In2 : Inport  Port=2
  mul_Dot Product3_dotp_0 : Product  Inputs=**  OutDataTypeStr=single  SampleTime=6.02409638554217e-09
  mul_Dot Product3_dotp_0_pd1 : Delay  DelayLength=6
  Out1 : Outport
  wires:
  In1/1 -> mul_Dot Product3_dotp_0/1
  In2/1 -> mul_Dot Product3_dotp_0/2
  mul_Dot Product3_dotp_0/1 -> mul_Dot Product3_dotp_0_pd1/1
  mul_Dot Product3_dotp_0_pd1/1 -> Out1/1

== system gm_MATE_HDLsolver_myFirstCircuit/ForFPGA/mul_Dot Product3_dotp_1 ==
  In1 : Inport
  In2 : Inport  Port=2
  mul_Dot Product3_dotp_1 : Product  Inputs=**  OutDataTypeStr=single  SampleTime=6.02409638554217e-09
  mul_Dot Product3_dotp_1_pd1 : Delay  DelayLength=6
  Out1 : Outport
  wires:
  In1/1 -> mul_Dot Product3_dotp_1/1
  In2/1 -> mul_Dot Product3_dotp_1/2
  mul_Dot Product3_dotp_1/1 -> mul_Dot Product3_dotp_1_pd1/1
  mul_Dot Product3_dotp_1_pd1/1 -> Out1/1

== system gm_MATE_HDLsolver_myFirstCircuit/ForFPGA/mul_Dot Product3_dotp_10 ==
  In1 : Inport
  In2 : Inport  Port=2
  mul_Dot Product3_dotp_10 : Product  Inputs=**  OutDataTypeStr=single  SampleTime=6.02409638554217e-09
  mul_Dot Product3_dotp_10_pd1 : Delay  DelayLength=6
  Out1 : Outport
  wires:
  In1/1 -> mul_Dot Product3_dotp_10/1
  In2/1 -> mul_Dot Product3_dotp_10/2
  mul_Dot Product3_dotp_10/1 -> mul_Dot Product3_dotp_10_pd1/1
  mul_Dot Product3_dotp_10_pd1/1 -> Out1/1

== system gm_MATE_HDLsolver_myFirstCircuit/ForFPGA/mul_Dot Product3_dotp_11 ==
  In1 : Inport
  In2 : Inport  Port=2
  mul_Dot Product3_dotp_11 : Product  Inputs=**  OutDataTypeStr=single  SampleTime=6.02409638554217e-09
  mul_Dot Product3_dotp_11_pd1 : Delay  DelayLength=6
  Out1 : Outport
  wires:
  In1/1 -> mul_Dot Product3_dotp_11/1
  In2/1 -> mul_Dot Product3_dotp_11/2
  mul_Dot Product3_dotp_11/1 -> mul_Dot Product3_dotp_11_pd1/1
  mul_Dot Product3_dotp_11_pd1/1 -> Out1/1

== system gm_MATE_HDLsolver_myFirstCircuit/ForFPGA/mul_Dot Product3_dotp_12 ==
  In1 : Inport
  In2 : Inport  Port=2
  mul_Dot Product3_dotp_12 : Product  Inputs=**  OutDataTypeStr=single  SampleTime=6.02409638554217e-09
  mul_Dot Product3_dotp_12_pd1 : Delay  DelayLength=6
  Out1 : Outport
  wires:
  In1/1 -> mul_Dot Product3_dotp_12/1
  In2/1 -> mul_Dot Product3_dotp_12/2
  mul_Dot Product3_dotp_12/1 -> mul_Dot Product3_dotp_12_pd1/1
  mul_Dot Product3_dotp_12_pd1/1 -> Out1/1

== system gm_MATE_HDLsolver_myFirstCircuit/ForFPGA/mul_Dot Product3_dotp_13 ==
  In1 : Inport
  In2 : Inport  Port=2
  mul_Dot Product3_dotp_13 : Product  Inputs=**  OutDataTypeStr=single  SampleTime=6.02409638554217e-09
  mul_Dot Product3_dotp_13_pd1 : Delay  DelayLength=6
  Out1 : Outport
  wires:
  In1/1 -> mul_Dot Product3_dotp_13/1
  In2/1 -> mul_Dot Product3_dotp_13/2
  mul_Dot Product3_dotp_13/1 -> mul_Dot Product3_dotp_13_pd1/1
  mul_Dot Product3_dotp_13_pd1/1 -> Out1/1

== system gm_MATE_HDLsolver_myFirstCircuit/ForFPGA/mul_Dot Product3_dotp_14 ==
  In1 : Inport
  In2 : Inport  Port=2
  mul_Dot Product3_dotp_14 : Product  Inputs=**  OutDataTypeStr=single  SampleTime=6.02409638554217e-09
  mul_Dot Product3_dotp_14_pd1 : Delay  DelayLength=6
  Out1 : Outport
  wires:
  In1/1 -> mul_Dot Product3_dotp_14/1
  In2/1 -> mul_Dot Product3_dotp_14/2
  mul_Dot Product3_dotp_14/1 -> mul_Dot Product3_dotp_14_pd1/1
  mul_Dot Product3_dotp_14_pd1/1 -> Out1/1

== system gm_MATE_HDLsolver_myFirstCircuit/ForFPGA/mul_Dot Product3_dotp_15 ==
  In1 : Inport
  In2 : Inport  Port=2
  mul_Dot Product3_dotp_15 : Product  Inputs=**  OutDataTypeStr=single  SampleTime=6.02409638554217e-09
  mul_Dot Product3_dotp_15_pd1 : Delay  DelayLength=6
  Out1 : Outport
  wires:
  In1/1 -> mul_Dot Product3_dotp_15/1
  In2/1 -> mul_Dot Product3_dotp_15/2
  mul_Dot Product3_dotp_15/1 -> mul_Dot Product3_dotp_15_pd1/1
  mul_Dot Product3_dotp_15_pd1/1 -> Out1/1

== system gm_MATE_HDLsolver_myFirstCircuit/ForFPGA/mul_Dot Product3_dotp_2 ==
  In1 : Inport
  In2 : Inport  Port=2
  mul_Dot Product3_dotp_2 : Product  Inputs=**  OutDataTypeStr=single  SampleTime=6.02409638554217e-09
  mul_Dot Product3_dotp_2_pd1 : Delay  DelayLength=6
  Out1 : Outport
  wires:
  In1/1 -> mul_Dot Product3_dotp_2/1
  In2/1 -> mul_Dot Product3_dotp_2/2
  mul_Dot Product3_dotp_2/1 -> mul_Dot Product3_dotp_2_pd1/1
  mul_Dot Product3_dotp_2_pd1/1 -> Out1/1

== system gm_MATE_HDLsolver_myFirstCircuit/ForFPGA/mul_Dot Product3_dotp_3 ==
  In1 : Inport
  In2 : Inport  Port=2
  mul_Dot Product3_dotp_3 : Product  Inputs=**  OutDataTypeStr=single  SampleTime=6.02409638554217e-09
  mul_Dot Product3_dotp_3_pd1 : Delay  DelayLength=6
  Out1 : Outport
  wires:
  In1/1 -> mul_Dot Product3_dotp_3/1
  In2/1 -> mul_Dot Product3_dotp_3/2
  mul_Dot Product3_dotp_3/1 -> mul_Dot Product3_dotp_3_pd1/1
  mul_Dot Product3_dotp_3_pd1/1 -> Out1/1

== system gm_MATE_HDLsolver_myFirstCircuit/ForFPGA/mul_Dot Product3_dotp_4 ==
  In1 : Inport
  In2 : Inport  Port=2
  mul_Dot Product3_dotp_4 : Product  Inputs=**  OutDataTypeStr=single  SampleTime=6.02409638554217e-09
  mul_Dot Product3_dotp_4_pd1 : Delay  DelayLength=6
  Out1 : Outport
  wires:
  In1/1 -> mul_Dot Product3_dotp_4/1
  In2/1 -> mul_Dot Product3_dotp_4/2
  mul_Dot Product3_dotp_4/1 -> mul_Dot Product3_dotp_4_pd1/1
  mul_Dot Product3_dotp_4_pd1/1 -> Out1/1

== system gm_MATE_HDLsolver_myFirstCircuit/ForFPGA/mul_Dot Product3_dotp_5 ==
  In1 : Inport
  In2 : Inport  Port=2
  mul_Dot Product3_dotp_5 : Product  Inputs=**  OutDataTypeStr=single  SampleTime=6.02409638554217e-09
  mul_Dot Product3_dotp_5_pd1 : Delay  DelayLength=6
  Out1 : Outport
  wires:
  In1/1 -> mul_Dot Product3_dotp_5/1
  In2/1 -> mul_Dot Product3_dotp_5/2
  mul_Dot Product3_dotp_5/1 -> mul_Dot Product3_dotp_5_pd1/1
  mul_Dot Product3_dotp_5_pd1/1 -> Out1/1

== system gm_MATE_HDLsolver_myFirstCircuit/ForFPGA/mul_Dot Product3_dotp_6 ==
  In1 : Inport
  In2 : Inport  Port=2
  mul_Dot Product3_dotp_6 : Product  Inputs=**  OutDataTypeStr=single  SampleTime=6.02409638554217e-09
  mul_Dot Product3_dotp_6_pd1 : Delay  DelayLength=6
  Out1 : Outport
  wires:
  In1/1 -> mul_Dot Product3_dotp_6/1
  In2/1 -> mul_Dot Product3_dotp_6/2
  mul_Dot Product3_dotp_6/1 -> mul_Dot Product3_dotp_6_pd1/1
  mul_Dot Product3_dotp_6_pd1/1 -> Out1/1

== system gm_MATE_HDLsolver_myFirstCircuit/ForFPGA/mul_Dot Product3_dotp_7 ==
  In1 : Inport
  In2 : Inport  Port=2
  mul_Dot Product3_dotp_7 : Product  Inputs=**  OutDataTypeStr=single  SampleTime=6.02409638554217e-09
  mul_Dot Product3_dotp_7_pd1 : Delay  DelayLength=6
  Out1 : Outport
  wires:
  In1/1 -> mul_Dot Product3_dotp_7/1
  In2/1 -> mul_Dot Product3_dotp_7/2
  mul_Dot Product3_dotp_7/1 -> mul_Dot Product3_dotp_7_pd1/1
  mul_Dot Product3_dotp_7_pd1/1 -> Out1/1

== system gm_MATE_HDLsolver_myFirstCircuit/ForFPGA/mul_Dot Product3_dotp_8 ==
  In1 : Inport
  In2 : Inport  Port=2
  mul_Dot Product3_dotp_8 : Product  Inputs=**  OutDataTypeStr=single  SampleTime=6.02409638554217e-09
  mul_Dot Product3_dotp_8_pd1 : Delay  DelayLength=6
  Out1 : Outport
  wires:
  In1/1 -> mul_Dot Product3_dotp_8/1
  In2/1 -> mul_Dot Product3_dotp_8/2
  mul_Dot Product3_dotp_8/1 -> mul_Dot Product3_dotp_8_pd1/1
  mul_Dot Product3_dotp_8_pd1/1 -> Out1/1

== system gm_MATE_HDLsolver_myFirstCircuit/ForFPGA/mul_Dot Product3_dotp_9 ==
  In1 : Inport
  In2 : Inport  Port=2
  mul_Dot Product3_dotp_9 : Product  Inputs=**  OutDataTypeStr=single  SampleTime=6.02409638554217e-09
  mul_Dot Product3_dotp_9_pd1 : Delay  DelayLength=6
  Out1 : Outport
  wires:
  In1/1 -> mul_Dot Product3_dotp_9/1
  In2/1 -> mul_Dot Product3_dotp_9/2
  mul_Dot Product3_dotp_9/1 -> mul_Dot Product3_dotp_9_pd1/1
  mul_Dot Product3_dotp_9_pd1/1 -> Out1/1

== system gm_MATE_HDLsolver_myFirstCircuit/ForFPGA/mul_Dot Product4_dotp_0 ==
  In1 : Inport
  In2 : Inport  Port=2
  mul_Dot Product4_dotp_0 : Product  Inputs=**  OutDataTypeStr=single  SampleTime=6.02409638554217e-09
  mul_Dot Product4_dotp_0_pd1 : Delay  DelayLength=6
  Out1 : Outport
  wires:
  In1/1 -> mul_Dot Product4_dotp_0/1
  In2/1 -> mul_Dot Product4_dotp_0/2
  mul_Dot Product4_dotp_0/1 -> mul_Dot Product4_dotp_0_pd1/1
  mul_Dot Product4_dotp_0_pd1/1 -> Out1/1

== system gm_MATE_HDLsolver_myFirstCircuit/ForFPGA/mul_Dot Product4_dotp_1 ==
  In1 : Inport
  In2 : Inport  Port=2
  mul_Dot Product4_dotp_1 : Product  Inputs=**  OutDataTypeStr=single  SampleTime=6.02409638554217e-09
  mul_Dot Product4_dotp_1_pd1 : Delay  DelayLength=6
  Out1 : Outport
  wires:
  In1/1 -> mul_Dot Product4_dotp_1/1
  In2/1 -> mul_Dot Product4_dotp_1/2
  mul_Dot Product4_dotp_1/1 -> mul_Dot Product4_dotp_1_pd1/1
  mul_Dot Product4_dotp_1_pd1/1 -> Out1/1

== system gm_MATE_HDLsolver_myFirstCircuit/ForFPGA/mul_Dot Product4_dotp_10 ==
  In1 : Inport
  In2 : Inport  Port=2
  mul_Dot Product4_dotp_10 : Product  Inputs=**  OutDataTypeStr=single  SampleTime=6.02409638554217e-09
  mul_Dot Product4_dotp_10_pd1 : Delay  DelayLength=6
  Out1 : Outport
  wires:
  In1/1 -> mul_Dot Product4_dotp_10/1
  In2/1 -> mul_Dot Product4_dotp_10/2
  mul_Dot Product4_dotp_10/1 -> mul_Dot Product4_dotp_10_pd1/1
  mul_Dot Product4_dotp_10_pd1/1 -> Out1/1

== system gm_MATE_HDLsolver_myFirstCircuit/ForFPGA/mul_Dot Product4_dotp_11 ==
  In1 : Inport
  In2 : Inport  Port=2
  mul_Dot Product4_dotp_11 : Product  Inputs=**  OutDataTypeStr=single  SampleTime=6.02409638554217e-09
  mul_Dot Product4_dotp_11_pd1 : Delay  DelayLength=6
  Out1 : Outport
  wires:
  In1/1 -> mul_Dot Product4_dotp_11/1
  In2/1 -> mul_Dot Product4_dotp_11/2
  mul_Dot Product4_dotp_11/1 -> mul_Dot Product4_dotp_11_pd1/1
  mul_Dot Product4_dotp_11_pd1/1 -> Out1/1

== system gm_MATE_HDLsolver_myFirstCircuit/ForFPGA/mul_Dot Product4_dotp_12 ==
  In1 : Inport
  In2 : Inport  Port=2
  mul_Dot Product4_dotp_12 : Product  Inputs=**  OutDataTypeStr=single  SampleTime=6.02409638554217e-09
  mul_Dot Product4_dotp_12_pd1 : Delay  DelayLength=6
  Out1 : Outport
  wires:
  In1/1 -> mul_Dot Product4_dotp_12/1
  In2/1 -> mul_Dot Product4_dotp_12/2
  mul_Dot Product4_dotp_12/1 -> mul_Dot Product4_dotp_12_pd1/1
  mul_Dot Product4_dotp_12_pd1/1 -> Out1/1

== system gm_MATE_HDLsolver_myFirstCircuit/ForFPGA/mul_Dot Product4_dotp_13 ==
  In1 : Inport
  In2 : Inport  Port=2
  mul_Dot Product4_dotp_13 : Product  Inputs=**  OutDataTypeStr=single  SampleTime=6.02409638554217e-09
  mul_Dot Product4_dotp_13_pd1 : Delay  DelayLength=6
  Out1 : Outport
  wires:
  In1/1 -> mul_Dot Product4_dotp_13/1
  In2/1 -> mul_Dot Product4_dotp_13/2
  mul_Dot Product4_dotp_13/1 -> mul_Dot Product4_dotp_13_pd1/1
  mul_Dot Product4_dotp_13_pd1/1 -> Out1/1

== system gm_MATE_HDLsolver_myFirstCircuit/ForFPGA/mul_Dot Product4_dotp_14 ==
  In1 : Inport
  In2 : Inport  Port=2
  mul_Dot Product4_dotp_14 : Product  Inputs=**  OutDataTypeStr=single  SampleTime=6.02409638554217e-09
  mul_Dot Product4_dotp_14_pd1 : Delay  DelayLength=6
  Out1 : Outport
  wires:
  In1/1 -> mul_Dot Product4_dotp_14/1
  In2/1 -> mul_Dot Product4_dotp_14/2
  mul_Dot Product4_dotp_14/1 -> mul_Dot Product4_dotp_14_pd1/1
  mul_Dot Product4_dotp_14_pd1/1 -> Out1/1

== system gm_MATE_HDLsolver_myFirstCircuit/ForFPGA/mul_Dot Product4_dotp_15 ==
  In1 : Inport
  In2 : Inport  Port=2
  mul_Dot Product4_dotp_15 : Product  Inputs=**  OutDataTypeStr=single  SampleTime=6.02409638554217e-09
  mul_Dot Product4_dotp_15_pd1 : Delay  DelayLength=6
  Out1 : Outport
  wires:
  In1/1 -> mul_Dot Product4_dotp_15/1
  In2/1 -> mul_Dot Product4_dotp_15/2
  mul_Dot Product4_dotp_15/1 -> mul_Dot Product4_dotp_15_pd1/1
  mul_Dot Product4_dotp_15_pd1/1 -> Out1/1

== system gm_MATE_HDLsolver_myFirstCircuit/ForFPGA/mul_Dot Product4_dotp_2 ==
  In1 : Inport
  In2 : Inport  Port=2
  mul_Dot Product4_dotp_2 : Product  Inputs=**  OutDataTypeStr=single  SampleTime=6.02409638554217e-09
  mul_Dot Product4_dotp_2_pd1 : Delay  DelayLength=6
  Out1 : Outport
  wires:
  In1/1 -> mul_Dot Product4_dotp_2/1
  In2/1 -> mul_Dot Product4_dotp_2/2
  mul_Dot Product4_dotp_2/1 -> mul_Dot Product4_dotp_2_pd1/1
  mul_Dot Product4_dotp_2_pd1/1 -> Out1/1

== system gm_MATE_HDLsolver_myFirstCircuit/ForFPGA/mul_Dot Product4_dotp_3 ==
  In1 : Inport
  In2 : Inport  Port=2
  mul_Dot Product4_dotp_3 : Product  Inputs=**  OutDataTypeStr=single  SampleTime=6.02409638554217e-09
  mul_Dot Product4_dotp_3_pd1 : Delay  DelayLength=6
  Out1 : Outport
  wires:
  In1/1 -> mul_Dot Product4_dotp_3/1
  In2/1 -> mul_Dot Product4_dotp_3/2
  mul_Dot Product4_dotp_3/1 -> mul_Dot Product4_dotp_3_pd1/1
  mul_Dot Product4_dotp_3_pd1/1 -> Out1/1

== system gm_MATE_HDLsolver_myFirstCircuit/ForFPGA/mul_Dot Product4_dotp_4 ==
  In1 : Inport
  In2 : Inport  Port=2
  mul_Dot Product4_dotp_4 : Product  Inputs=**  OutDataTypeStr=single  SampleTime=6.02409638554217e-09
  mul_Dot Product4_dotp_4_pd1 : Delay  DelayLength=6
  Out1 : Outport
  wires:
  In1/1 -> mul_Dot Product4_dotp_4/1
  In2/1 -> mul_Dot Product4_dotp_4/2
  mul_Dot Product4_dotp_4/1 -> mul_Dot Product4_dotp_4_pd1/1
  mul_Dot Product4_dotp_4_pd1/1 -> Out1/1

== system gm_MATE_HDLsolver_myFirstCircuit/ForFPGA/mul_Dot Product4_dotp_5 ==
  In1 : Inport
  In2 : Inport  Port=2
  mul_Dot Product4_dotp_5 : Product  Inputs=**  OutDataTypeStr=single  SampleTime=6.02409638554217e-09
  mul_Dot Product4_dotp_5_pd1 : Delay  DelayLength=6
  Out1 : Outport
  wires:
  In1/1 -> mul_Dot Product4_dotp_5/1
  In2/1 -> mul_Dot Product4_dotp_5/2
  mul_Dot Product4_dotp_5/1 -> mul_Dot Product4_dotp_5_pd1/1
  mul_Dot Product4_dotp_5_pd1/1 -> Out1/1

== system gm_MATE_HDLsolver_myFirstCircuit/ForFPGA/mul_Dot Product4_dotp_6 ==
  In1 : Inport
  In2 : Inport  Port=2
  mul_Dot Product4_dotp_6 : Product  Inputs=**  OutDataTypeStr=single  SampleTime=6.02409638554217e-09
  mul_Dot Product4_dotp_6_pd1 : Delay  DelayLength=6
  Out1 : Outport
  wires:
  In1/1 -> mul_Dot Product4_dotp_6/1
  In2/1 -> mul_Dot Product4_dotp_6/2
  mul_Dot Product4_dotp_6/1 -> mul_Dot Product4_dotp_6_pd1/1
  mul_Dot Product4_dotp_6_pd1/1 -> Out1/1

== system gm_MATE_HDLsolver_myFirstCircuit/ForFPGA/mul_Dot Product4_dotp_7 ==
  In1 : Inport
  In2 : Inport  Port=2
  mul_Dot Product4_dotp_7 : Product  Inputs=**  OutDataTypeStr=single  SampleTime=6.02409638554217e-09
  mul_Dot Product4_dotp_7_pd1 : Delay  DelayLength=6
  Out1 : Outport
  wires:
  In1/1 -> mul_Dot Product4_dotp_7/1
  In2/1 -> mul_Dot Product4_dotp_7/2
  mul_Dot Product4_dotp_7/1 -> mul_Dot Product4_dotp_7_pd1/1
  mul_Dot Product4_dotp_7_pd1/1 -> Out1/1

== system gm_MATE_HDLsolver_myFirstCircuit/ForFPGA/mul_Dot Product4_dotp_8 ==
  In1 : Inport
  In2 : Inport  Port=2
  mul_Dot Product4_dotp_8 : Product  Inputs=**  OutDataTypeStr=single  SampleTime=6.02409638554217e-09
  mul_Dot Product4_dotp_8_pd1 : Delay  DelayLength=6
  Out1 : Outport
  wires:
  In1/1 -> mul_Dot Product4_dotp_8/1
  In2/1 -> mul_Dot Product4_dotp_8/2
  mul_Dot Product4_dotp_8/1 -> mul_Dot Product4_dotp_8_pd1/1
  mul_Dot Product4_dotp_8_pd1/1 -> Out1/1

== system gm_MATE_HDLsolver_myFirstCircuit/ForFPGA/mul_Dot Product4_dotp_9 ==
  In1 : Inport
  In2 : Inport  Port=2
  mul_Dot Product4_dotp_9 : Product  Inputs=**  OutDataTypeStr=single  SampleTime=6.02409638554217e-09
  mul_Dot Product4_dotp_9_pd1 : Delay  DelayLength=6
  Out1 : Outport
  wires:
  In1/1 -> mul_Dot Product4_dotp_9/1
  In2/1 -> mul_Dot Product4_dotp_9/2
  mul_Dot Product4_dotp_9/1 -> mul_Dot Product4_dotp_9_pd1/1
  mul_Dot Product4_dotp_9_pd1/1 -> Out1/1

== system gm_MATE_HDLsolver_myFirstCircuit/ForFPGA/mul_Dot Product5_dotp_0 ==
  In1 : Inport
  In2 : Inport  Port=2
  mul_Dot Product5_dotp_0 : Product  Inputs=**  OutDataTypeStr=single  SampleTime=6.02409638554217e-09
  mul_Dot Product5_dotp_0_pd1 : Delay  DelayLength=6
  Out1 : Outport
  wires:
  In1/1 -> mul_Dot Product5_dotp_0/1
  In2/1 -> mul_Dot Product5_dotp_0/2
  mul_Dot Product5_dotp_0/1 -> mul_Dot Product5_dotp_0_pd1/1
  mul_Dot Product5_dotp_0_pd1/1 -> Out1/1

== system gm_MATE_HDLsolver_myFirstCircuit/ForFPGA/mul_Dot Product5_dotp_1 ==
  In1 : Inport
  In2 : Inport  Port=2
  mul_Dot Product5_dotp_1 : Product  Inputs=**  OutDataTypeStr=single  SampleTime=6.02409638554217e-09
  mul_Dot Product5_dotp_1_pd1 : Delay  DelayLength=6
  Out1 : Outport
  wires:
  In1/1 -> mul_Dot Product5_dotp_1/1
  In2/1 -> mul_Dot Product5_dotp_1/2
  mul_Dot Product5_dotp_1/1 -> mul_Dot Product5_dotp_1_pd1/1
  mul_Dot Product5_dotp_1_pd1/1 -> Out1/1

== system gm_MATE_HDLsolver_myFirstCircuit/ForFPGA/mul_Dot Product5_dotp_10 ==
  In1 : Inport
  In2 : Inport  Port=2
  mul_Dot Product5_dotp_10 : Product  Inputs=**  OutDataTypeStr=single  SampleTime=6.02409638554217e-09
  mul_Dot Product5_dotp_10_pd1 : Delay  DelayLength=6
  Out1 : Outport
  wires:
  In1/1 -> mul_Dot Product5_dotp_10/1
  In2/1 -> mul_Dot Product5_dotp_10/2
  mul_Dot Product5_dotp_10/1 -> mul_Dot Product5_dotp_10_pd1/1
  mul_Dot Product5_dotp_10_pd1/1 -> Out1/1
